simulink model "inverter_subsystem"  (R2022b)
settings: Solver=ode45  StartTime=0.0  StopTime=10.0  RelTol=1e-3  EnableMultiTasking=on
libraries: spsIGBTDiodeLib x8, simulink x4, spsDCVoltageSourceLib x2, spsCurrentMeasurementLib x1, spsSeriesRLCBranchLib x1, spsTHDLib x1, spsVoltageMeasurementLib x1, spspowerguiLib x1
settings Model: Creator=ugoch  LastModifiedBy=ugochukwu
settings SolverCC: AlgebraicLoopSolver=TrustRegion
settings DataIOCC: LimitDataPoints=on  SaveFormat=Array  ReturnWorkspaceOutputs=off
settings OptimizationCC: LifeSpan=inf
settings DebuggingCC: SolverPrmCheckMsg=warning  UnconnectedInputMsg=warning  UnconnectedOutputMsg=warning  UnconnectedLineMsg=warning  SFUnexpectedBacktrackingDiag=warning  SFNoUnconditionalDefaultTransitionDiag=warning  SFExecutionAtInitializationDiag=none  SFMachineParentedDataDiag=warning  ArithmeticOperatorsInVariantConditions=warning
settings HardwareCC: ProdBitPerPointer=32  ProdBitPerSizeT=32  ProdBitPerPtrDiffT=32  ProdLargestAtomicFloat=None  ProdIntDivRoundTo=Undefined  ProdEndianess=Unspecified  ProdWordSize=32  ProdHWDeviceType=32-bit Generic
settings ModelReferenceCC: PropagateSignalLabelsOutOfModel=off
settings SFSimCC: SimUseLocalCustomCode=off  CustomCodeUndefinedFunction=UseInterfaceOnly
settings RTWCC: RTWUseLocalCustomCode=off
settings CodeAppCC: StateflowObjectComments=on
settings GRTTargetCC: TargetLangStandard=C89/C90 (ANSI)
settings ConfigComp: CovMetricSettings=dw  CovSaveCumulativeToWorkspaceVar=on  CovSaveSingleToWorkspaceVar=on  CovExternalEMLEnable=off  CovSFcnEnable=off
settings SimscapeCC: SimscapeNormalizeSystem=off

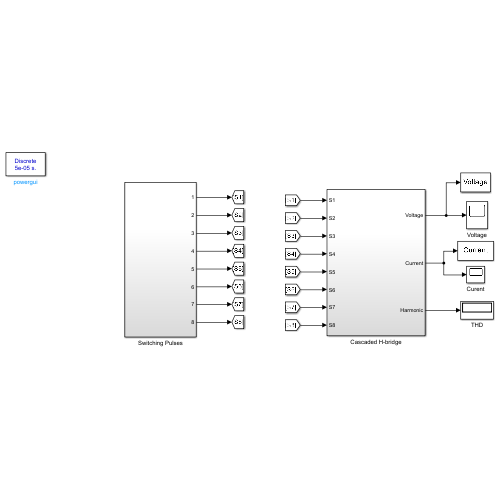
[thumbnail: Simulink's stored preview of the top-level diagram]
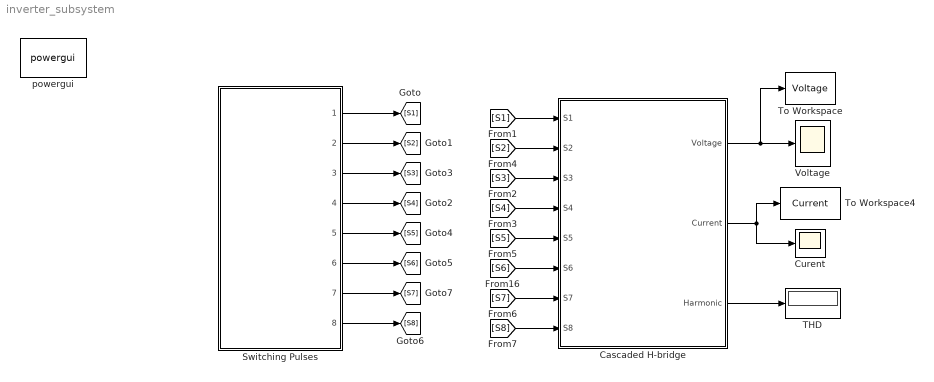
== system inverter_subsystem ==
  Cascaded H-bridge : Subsystem
  Curent : Scope
  Switching Pulses : Subsystem
  THD : Display
  To Workspace : ToWorkspace  VariableName=Voltage  SaveFormat=Timeseries  SampleTime=-1
  To Workspace4 : ToWorkspace  VariableName=Current  SaveFormat=Timeseries  SampleTime=-1
  Voltage : Scope
  powergui : spspowerguiLib/powergui  Priority=1  SimulationMode=Discrete  SampleTime=50e-6  frequency=60  Iterations=50  frequencyindice=0  Pbase=100e6  ErrMax=1e-4  UnitsV=kV  UnitsW=MW  buscounter=0  FunctionMessages=off  echomessages=off  EnableUseOfTLC=off  CurrentSourceSwitches=off  DisableSnubberDevices=off  DisableRonSwitches=off  DisableVfSwitches=off  DisplayEquations=off  AutomaticDiscreteSolvers=off  SolverType=Tustin  Interpol=off  ExternalGateDelay=off  methode=off  Ts=0  x0status=blocks  SPID=off  SwTol=0  HookPort=off  NonlinearTolerance=1e-4  nMaxIteration=100  ContinueOnMaxIteration=off  RestoreLinks=warning  ResistiveCurrentMeasurement=off  Frange=[0:2:500]  Ylog=off  Xlog=on  ShowGrid=off  save=off  variable=ZData  structure=0  ZoomFFT=off  StartTime=0.0  cycles=1  DisplayStyle=1  fundamental=60  FreqAxis=off  MaxFrequency=1000  frequencyindicesteady=1  RmsSteady=1  display=off
  wires:
  Switching Pulses/1(1) -> [S1]
  Switching Pulses/2(2) -> [S2]
  Switching Pulses/3(3) -> [S3]
  Switching Pulses/4(4) -> [S4]
  Switching Pulses/5(5) -> [S5]
  Switching Pulses/6(6) -> [S6]
  Switching Pulses/7(7) -> [S7]
  Switching Pulses/8(8) -> [S8]
  [S1] -> Cascaded H-bridge/1(S1)
  [S2] -> Cascaded H-bridge/2(S2)
  [S3] -> Cascaded H-bridge/3(S3)
  [S4] -> Cascaded H-bridge/4(S4)
  [S5] -> Cascaded H-bridge/5(S5)
  [S6] -> Cascaded H-bridge/6(S6)
  [S7] -> Cascaded H-bridge/7(S7)
  [S8] -> Cascaded H-bridge/8(S8)
  Cascaded H-bridge/2(Current) -> Curent/1, To Workspace4/1
  Cascaded H-bridge/1(Voltage) -> To Workspace/1, Voltage/1
  Cascaded H-bridge/3(Harmonic) -> THD/1

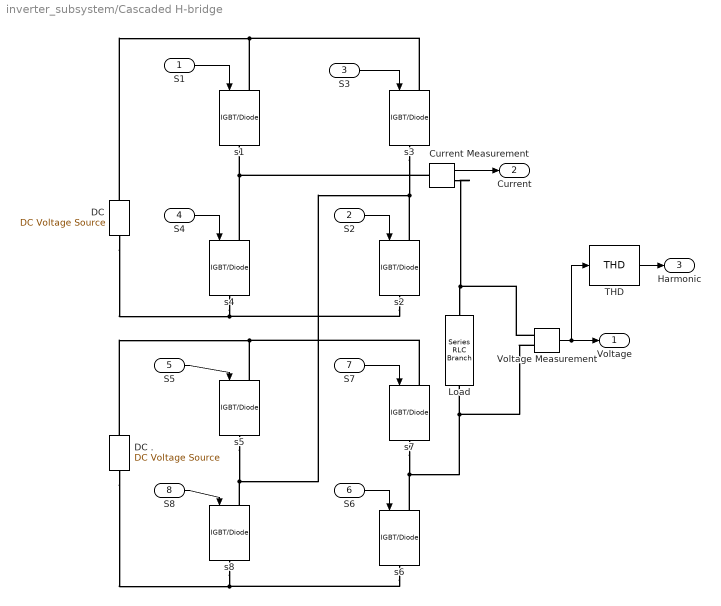
== system inverter_subsystem/Cascaded H-bridge ==
  S1 : Inport
  S2 : Inport  Port=2
  S3 : Inport  Port=3
  S4 : Inport  Port=4
  S5 : Inport  Port=5
  S6 : Inport  Port=6
  S7 : Inport  Port=7
  S8 : Inport  Port=8
  Current Measurement : spsCurrentMeasurementLib/Current Measurement  PhasorSimulation=off  OutputType=Complex  PSBequivalent=0
  DC : spsDCVoltageSourceLib/DC Voltage Source  Amplitude=110  Measurements=None
  DC . : spsDCVoltageSourceLib/DC Voltage Source  Amplitude=110  Measurements=None
  Load : spsSeriesRLCBranchLib/Series RLC Branch  LConnTagsString=__new0  RConnTagsString=__new0  BranchType=RL  Resistance=1  Inductance=1e-3  SetiL0=off  InitialCurrent=0  Capacitance=1e-6  Setx0=off  InitialVoltage=0  Measurements=None
  THD : spsTHDLib/THD  Freq=50  Ts=0
  Voltage Measurement : spsVoltageMeasurementLib/Voltage Measurement  PhasorSimulation=off  OutputType=Complex  PSBequivalent=0
  s{1..8} (8 alike) : spsIGBTDiodeLib/IGBT//Diode  Ron=1e-3  Rs=1e5  Cs=inf  Measurements=off
  Voltage : Outport
  Current : Outport  Port=2
  Harmonic : Outport  Port=3
  wires:
  S1/1 -> s1/1
  S3/1 -> s3/1
  S5/1 -> s5/1
  S8/1 -> s8/1
  S4/1 -> s4/1
  Voltage Measurement/1 -> THD/1, Voltage/1
  S7/1 -> s7/1
  S6/1 -> s6/1
  S2/1 -> s2/1
  Current Measurement/1 -> Current/1
  THD/1 -> Harmonic/1
  connections:
  s1/LConn1 -- s3/LConn1 -- DC/RConn1
  s5/LConn1 -- s7/LConn1 -- DC ./RConn1
  Voltage Measurement/LConn1 -- Current Measurement/RConn1 -- Load/RConn1
  DC/LConn1 -- s2/RConn1 -- s4/RConn1
  s2/LConn1 -- s5/RConn1 -- s8/LConn1 -- s3/RConn1
  DC ./LConn1 -- s6/RConn1 -- s8/RConn1
  Load/LConn1 -- s6/LConn1 -- s7/RConn1 -- Voltage Measurement/LConn2
  s4/LConn1 -- Current Measurement/LConn1 -- s1/RConn1

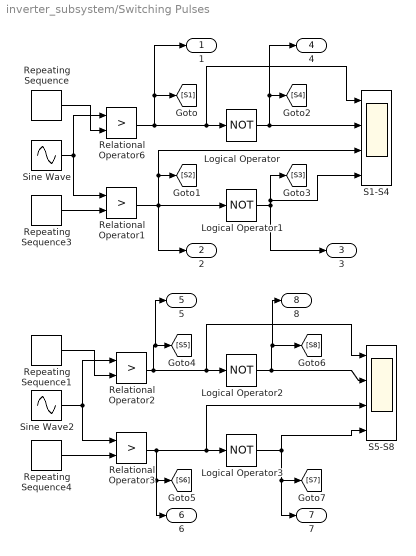
== system inverter_subsystem/Switching Pulses ==
  Logical Operator{,1..3} (4 alike) : Logic  Operator=NOT  AllPortsSameDT=off  OutDataTypeStr=boolean
  Relational Operator{1..3,6} (4 alike) : RelationalOperator  Operator=>  OutDataTypeStr=boolean  InputSameDT=off
  Repeating Sequence : simulink/Sources/Repeating Sequence  rep_seq_t=[0 1/4000 1/2000]  rep_seq_y=[1 1.5 1 ]
  Repeating Sequence1 : simulink/Sources/Repeating Sequence  rep_seq_t=[0 1/4000 1/2000]  rep_seq_y=[0.5 1 0.5]
  Repeating Sequence3 : simulink/Sources/Repeating Sequence  rep_seq_t=[0 1/4000 1/2000]  rep_seq_y=[-1.5 -1 -1.5 ]
  Repeating Sequence4 : simulink/Sources/Repeating Sequence  rep_seq_t=[0 1/4000 1/2000]  rep_seq_y=[-1 -0.5 -1]
  S1-S4 : Scope  NumInputPorts=4
  S5-S8 : Scope  NumInputPorts=4
  Sine Wave : Sin  Amplitude=1.4  Frequency=2*50*pi  SampleTime=0
  Sine Wave2 : Sin  Amplitude=1.4  Frequency=2*50*pi  SampleTime=0
  1 : Outport
  2 : Outport  Port=2
  3 : Outport  Port=3
  4 : Outport  Port=4
  5 : Outport  Port=5
  6 : Outport  Port=6
  7 : Outport  Port=7
  8 : Outport  Port=8
  wires:
  Logical Operator1/1 -> 3/1, [S3], S1-S4/4
  Relational Operator2/1 -> Logical Operator2/1, S5-S8/1, 5/1, [S5]
  Relational Operator1/1 -> 2/1, S1-S4/3, [S2], Logical Operator1/1
  Relational Operator3/1 -> Logical Operator3/1, S5-S8/3, 6/1, [S6]
  Logical Operator3/1 -> 7/1, [S7], S5-S8/4
  Sine Wave/1 -> Relational Operator6/1, Relational Operator1/1
  Repeating Sequence/1 -> Relational Operator6/2
  Sine Wave2/1 -> Relational Operator2/1, Relational Operator3/1
  Relational Operator6/1 -> Logical Operator/1, S1-S4/1, 1/1, [S1]
  Repeating Sequence1/1 -> Relational Operator2/2
  Repeating Sequence4/1 -> Relational Operator3/2
  Repeating Sequence3/1 -> Relational Operator1/2
  Logical Operator/1 -> S1-S4/2, 4/1, [S4]
  Logical Operator2/1 -> S5-S8/2, 8/1, [S8]
